simulink model "bob_est_sim"  (R2024a)
settings: Solver=VariableStepAuto  StartTime=0.0  StopTime=20  RelTol=1e-3
values from neighbouring files (symbols this model uses):
  A = eye(size(A)) + Ts * A    [bob_est_ini.m]
  Ae = [[A, B]; [0, 0, 1]]    [bob_est_ini.m]
  B = Ts * B    [bob_est_ini.m]
  Be = [B; 0]    [bob_est_ini.m]
  C = [1 0]    [bob_est_ini.m]
  Ce = [C, 0]    [bob_est_ini.m]
  K = dlqr(A.', C.', Q, R).'    [bob_est_ini.m]
  Ke = dlqr(Ae.', Ce.', Qe, R).'    [bob_est_ini.m]
  Ts = 1e-3    (= 0.001)    [bob_est_ini.m]
libraries: cstblocks x3, simulink x1
settings Model: Creator=miche  LastModifiedBy=miche

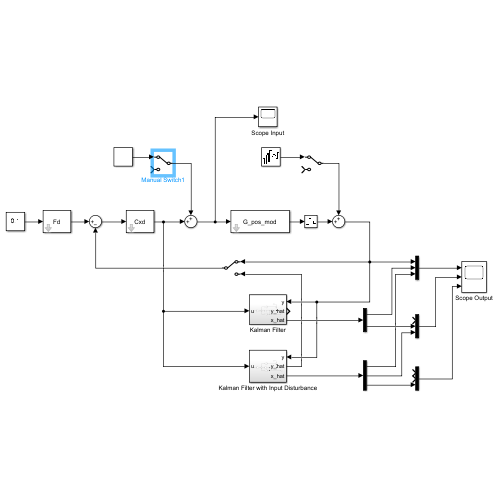
[thumbnail: Simulink's stored preview of the top-level diagram]
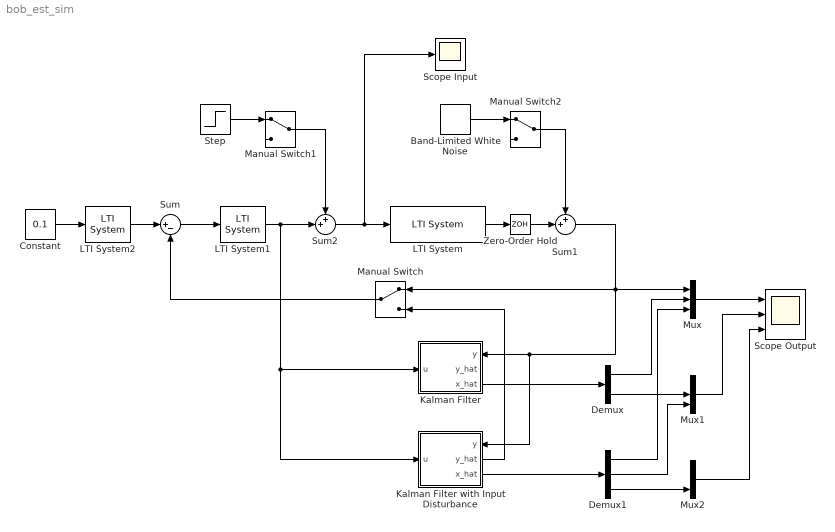
== system bob_est_sim ==
  Band-Limited White Noise : simulink/Sources/Band-Limited White Noise  Cov=1e-9  Ts=Ts  seed=[23341]
  Constant : Constant  Value=0.1
  Demux : Demux  Outputs=2
  Demux1 : Demux  Outputs=3
  Kalman Filter : Subsystem
      settings: PortSchema="{\"entries\":[{\"content\":{\"sides\":[{\"content\":{\"connectorIds\":[\"In1\"]},\"type\":\"ConnectorPlacement.EquallySpacedRectSide\",\"uuid\":\"dbb87334-7e66-45de-a50d-945c362a882e\"},{\"content\":{\"connectorIds\":[\"In2\",\"Out1\",\"Out2\"],\"side\":\"RIGHT\"},\"type\":\"ConnectorPlacement.EquallySpacedRectSide\",\"uuid\":\"b0a8b261-aa93-4baf-b8e5-3abd1e39c584\"},{\"content\":{\"side\":\"TOP\"},\"type\":\"ConnectorPlacement.EquallySpacedRectSide\",\"uuid\":\"509a5763-1d94-41fb-a38b-7cbe309d9921\"}]},\"type\":\"ConnectorPlacement.EquallySpacedConnector\",\"uuid\":\"bfdf310b-0ec8-4e23-8eba-2069b07672d5\"}],\"packageUris\":[\"http://schema.mathworks.com/mf0/Connector/R2020b\"],\"version\":\"1.0\"}"
  Kalman Filter with Input Disturbance : Subsystem
      settings: PortSchema="{\"entries\":[{\"content\":{\"sides\":[{\"content\":{\"connectorIds\":[\"In1\"]},\"type\":\"ConnectorPlacement.EquallySpacedRectSide\",\"uuid\":\"dbb87334-7e66-45de-a50d-945c362a882e\"},{\"content\":{\"connectorIds\":[\"In2\",\"Out1\",\"Out2\"],\"side\":\"RIGHT\"},\"type\":\"ConnectorPlacement.EquallySpacedRectSide\",\"uuid\":\"b0a8b261-aa93-4baf-b8e5-3abd1e39c584\"},{\"content\":{\"side\":\"TOP\"},\"type\":\"ConnectorPlacement.EquallySpacedRectSide\",\"uuid\":\"509a5763-1d94-41fb-a38b-7cbe309d9921\"}]},\"type\":\"ConnectorPlacement.EquallySpacedConnector\",\"uuid\":\"bfdf310b-0ec8-4e23-8eba-2069b07672d5\"}],\"packageUris\":[\"http://schema.mathworks.com/mf0/Connector/R2020b\"],\"version\":\"1.0\"}"
  LTI System : cstblocks/LTI System  sys=G_pos_mod  IC=[]  PadeOrder=0
  LTI System1 : cstblocks/LTI System  sys=Cxd  IC=[]  PadeOrder=0
  LTI System2 : cstblocks/LTI System  sys=Fd  IC=[]  PadeOrder=0
  Manual Switch : ManualSwitch
  Manual Switch1 : ManualSwitch
  Manual Switch2 : ManualSwitch
  Mux : Mux  Inputs=3
  Mux1 : Mux  Inputs=3
  Mux2 : Mux  Inputs=3
  Scope Input : Scope
  Scope Output : Scope  NumInputPorts=3
  Step : Step  Time=6  After=0.01  SampleTime=0
  Sum : Sum  Inputs=|+-
  Sum1 : Sum  Inputs=++|
  Sum2 : Sum  Inputs=++|
  Zero-Order Hold : ZeroOrderHold  SampleTime=Ts
  wires:
  LTI System1/1 -> Sum2/2, Kalman Filter with Input Disturbance/1(u), Kalman Filter/1(u)
  Constant/1 -> LTI System2/1
  LTI System/1 -> Zero-Order Hold/1
  Sum1/1 -> Manual Switch/1, Kalman Filter with Input Disturbance/2(y), Kalman Filter/2(y), Mux/1
  Sum/1 -> LTI System1/1
  LTI System2/1 -> Sum/1
  Kalman Filter/2(x_hat) -> Demux/1
  Zero-Order Hold/1 -> Sum1/2
  Demux/1 -> Mux/2
  Demux/2 -> Mux1/2
  Mux/1 -> Scope Output/1
  Mux1/1 -> Scope Output/2
  Sum2/1 -> Scope Input/1, LTI System/1
  Kalman Filter with Input Disturbance/2(x_hat) -> Demux1/1
  Demux1/1 -> Mux/3
  Demux1/2 -> Mux1/3
  Demux1/3 -> Mux2/3
  Mux2/1 -> Scope Output/3
  Kalman Filter with Input Disturbance/1(y_hat) -> Manual Switch/2
  Manual Switch/1 -> Sum/2
  Step/1 -> Manual Switch1/1
  Manual Switch1/1 -> Sum2/1
  Band-Limited White Noise/1 -> Manual Switch2/1
  Manual Switch2/1 -> Sum1/1

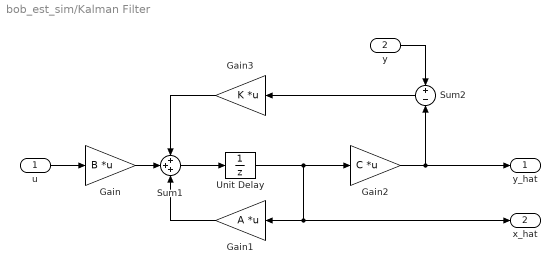
== system bob_est_sim/Kalman Filter ==
  u : Inport
  y : Inport  Port=2
  Gain : Gain  Gain=B  Multiplication=Matrix(K*u)
  Gain1 : Gain  Gain=A  Multiplication=Matrix(K*u)
  Gain2 : Gain  Gain=C  Multiplication=Matrix(K*u)
  Gain3 : Gain  Gain=K  Multiplication=Matrix(K*u)
  Sum1 : Sum  Inputs=+++
  Sum2 : Sum  Inputs=+|-
  Unit Delay : UnitDelay  SampleTime=Ts  HasFrameUpgradeWarning=on
  y_hat : Outport
  x_hat : Outport  Port=2
  wires:
  Gain/1 -> Sum1/2
  u/1 -> Gain/1
  Gain1/1 -> Sum1/3
  Gain2/1 -> y_hat/1, Sum2/2
  Unit Delay/1 -> Gain2/1, x_hat/1, Gain1/1
  Sum1/1 -> Unit Delay/1
  Sum2/1 -> Gain3/1
  Gain3/1 -> Sum1/1
  y/1 -> Sum2/1

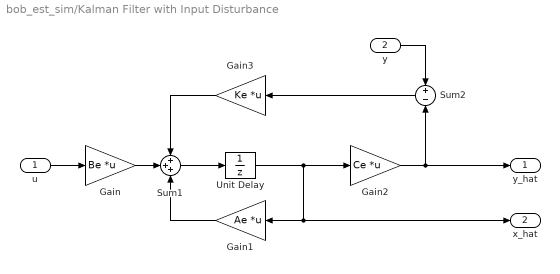
== system bob_est_sim/Kalman Filter with Input Disturbance ==
  u : Inport
  y : Inport  Port=2
  Gain : Gain  Gain=Be  Multiplication=Matrix(K*u)
  Gain1 : Gain  Gain=Ae  Multiplication=Matrix(K*u)
  Gain2 : Gain  Gain=Ce  Multiplication=Matrix(K*u)
  Gain3 : Gain  Gain=Ke  Multiplication=Matrix(K*u)
  Sum1 : Sum  Inputs=+++
  Sum2 : Sum  Inputs=+|-
  Unit Delay : UnitDelay  SampleTime=Ts  HasFrameUpgradeWarning=on
  y_hat : Outport
  x_hat : Outport  Port=2
  wires:
  y/1 -> Sum2/1
  Gain3/1 -> Sum1/1
  Sum2/1 -> Gain3/1
  Sum1/1 -> Unit Delay/1
  Unit Delay/1 -> Gain1/1, x_hat/1, Gain2/1
  Gain2/1 -> Sum2/2, y_hat/1
  Gain1/1 -> Sum1/3
  u/1 -> Gain/1
  Gain/1 -> Sum1/2
